simulink model "finalproject"  (R2022a)
settings: Solver=VariableStepAuto  StartTime=0.0  StopTime=0.1  RelTol=1e-3
values from neighbouring files (symbols this model uses):
  A_opamp = 2e5    (= 200000)    [flybackcode.m]
  C = 5e-3    (= 0.005)    [flybackcode.m]
  C1 = 25.6e-9    (= 2.56e-08)    [flybackcode.m]
  C2 = 3.02e-9    (= 3.02e-09)    [flybackcode.m]
  C3 = 4.4e-9    (= 4.4e-09)    [flybackcode.m]
  limit = 0.1    [flybackcode.m]
  R1 = 100e3    (= 100000)    [flybackcode.m]
  R2 = 18.918e3    (= 18918)    [flybackcode.m]
  R3 = 11.5e3    (= 11500)    [flybackcode.m]
  Ra = ((Vo/Vref) *Rb)- Rb    (= 400000)    [flybackcode.m]
  Rb = 100e3    (= 100000)    [flybackcode.m]
  Rin_opamp = 1e7    (= 10000000)    [flybackcode.m]
  RL = 2.05326    [flybackcode.m]
  Rout_opamp = 1e-3    (= 0.001)    [flybackcode.m]
  Vp = Vref/D    (= 5.90115564298)    [flybackcode.m]
  Vref = 2.4    [flybackcode.m]
libraries: spsSeriesRLCBranchLib x13, spsVoltageMeasurementLib x5, spsDCVoltageSourceLib x2, slctrlblks x1, spsCurrentMeasurementLib x1, spsDiodeLib x1, spsGroundLib x1, spsLinearTransformerLib x1, spsMosfetLib x1, spsSawtoothGeneratorLib x1, spsControlledVoltageSourceLib x1, spspowerguiLib x1
settings Model: Creator=justi  LastModifiedBy=justi

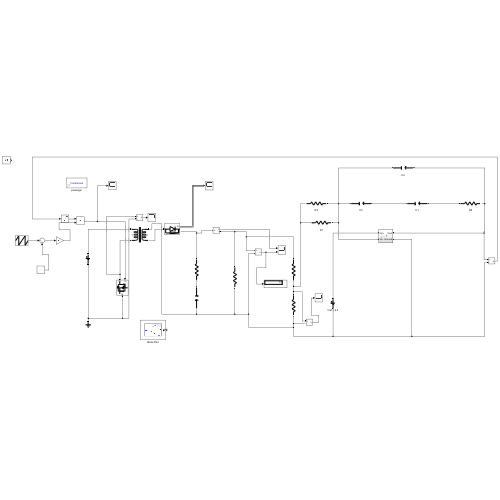
[thumbnail: Simulink's stored preview of the top-level diagram]
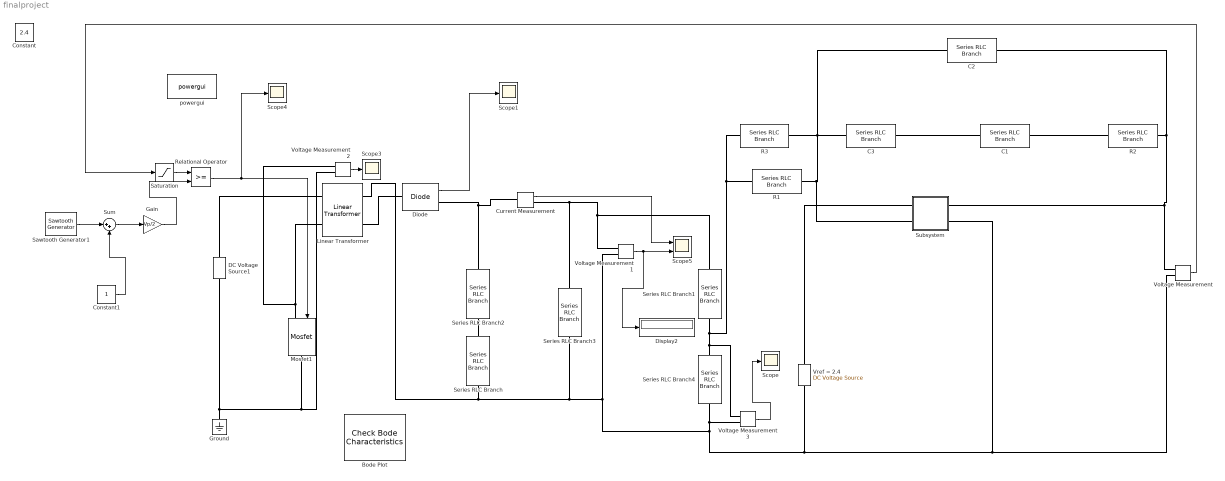
== system finalproject ==
  Bode Plot : slctrlblks/Model Verification/Check Bode  Characteristics  InstantiateOnLoad=on  SaveOperatingPoints=off  LinearizationIOs={'/Relational Operator', 1, 'in', 'off', '';'/Voltage Measurement1', 1, 'out', 'on', ''}  LinearizeAt=SnapshotTimes  SnapshotTimes=[0]  TriggerType=rising  SampleTime=auto  RateConversionMethod=zoh  PreWarpFreq=10  UseExactDelayModel=off  UseFullBlockNameLabels=off  UseBusSignalLabels=off  enabled=on  stopWhenAssertionFail=off  export=on  ViewDlgPos=[460 610 601 534]  OpenViewOnLoad=on  LaunchViewOnOpen=off  FrequencyUnits=rad/s  MagnitudeUnits=dB  PhaseUnits=deg  TimeUnits=seconds  EnableUpperBound=on  UpperBoundFrequencies=[]  UpperBoundMagnitudes=[]  EnableLowerBound=off  LowerBoundFrequencies=[]  LowerBoundMagnitudes=[]
      settings: SaveToWorkspace=on
  C1 : spsSeriesRLCBranchLib/Series RLC Branch  LConnTagsString=__new0  RConnTagsString=__new0  BranchType=C  Resistance=R3  Inductance=1e-3  SetiL0=off  InitialCurrent=0  Capacitance=C1  Setx0=off  InitialVoltage=0  Measurements=None
  C2 : spsSeriesRLCBranchLib/Series RLC Branch  LConnTagsString=__new0  RConnTagsString=__new0  BranchType=C  Resistance=R3  Inductance=1e-3  SetiL0=off  InitialCurrent=0  Capacitance=C2  Setx0=off  InitialVoltage=0  Measurements=None
  C3 : spsSeriesRLCBranchLib/Series RLC Branch  LConnTagsString=__new0  RConnTagsString=__new0  BranchType=C  Resistance=R3  Inductance=1e-3  SetiL0=off  InitialCurrent=0  Capacitance=C3  Setx0=off  InitialVoltage=0  Measurements=None
  Constant : Constant  Value=2.4
  Constant1 : Constant
  Current Measurement : spsCurrentMeasurementLib/Current Measurement  PhasorSimulation=off  OutputType=Complex  PSBequivalent=0
  DC Voltage Source1 : spsDCVoltageSourceLib/DC Voltage Source  Amplitude=70  Measurements=None
  Diode : spsDiodeLib/Diode  Ron=0.001  Lon=0  Vf=0.8  IC=0  UseSnubber=0  Rs=500  Cs=250e-9  Measurements=on
  Display2 : Display
  Gain : Gain  Gain=Vp/2
  Ground : spsGroundLib/Ground  LConnTagsString=a
  Linear Transformer : spsLinearTransformerLib/Linear Transformer  UNITS=SI  NominalPower=[ 250e6 100e3 ]  winding1=[280 0 0]  winding2=[70 0 0]  ThreeWindings=off  winding3=[3.15e+05 0.7938 0.084225]  RmLm=[1.0804e+05 100e-6]  Measurements=None  DataType=on
  Mosfet1 : spsMosfetLib/Mosfet  Ron=0.1  Lon=0  Rd=0  Vfd=0  IC=0  Rs=1e5  Cs=inf  Measurements=off
  R1 : spsSeriesRLCBranchLib/Series RLC Branch  LConnTagsString=__new0  RConnTagsString=__new0  BranchType=R  Resistance=R1  Inductance=1e-3  SetiL0=off  InitialCurrent=0  Capacitance=1e-6  Setx0=off  InitialVoltage=0  Measurements=None
  R2 : spsSeriesRLCBranchLib/Series RLC Branch  LConnTagsString=__new0  RConnTagsString=__new0  BranchType=R  Resistance=R2  Inductance=1e-3  SetiL0=off  InitialCurrent=0  Capacitance=1e-6  Setx0=off  InitialVoltage=0  Measurements=None
  R3 : spsSeriesRLCBranchLib/Series RLC Branch  LConnTagsString=__new0  RConnTagsString=__new0  BranchType=R  Resistance=R3  Inductance=1e-3  SetiL0=off  InitialCurrent=0  Capacitance=1e-6  Setx0=off  InitialVoltage=0  Measurements=None
  Relational Operator : RelationalOperator  OutDataTypeStr=boolean  RndMeth=Simplest  InputSameDT=off
  Saturation : Saturate  UpperLimit=Vp-limit  LowerLimit=0+limit
  Sawtooth Generator1 : spsSawtoothGeneratorLib/Sawtooth Generator  Freq=fsw  Phase=-180  Ts=0
  Scope{,1,3..4} (4 alike) : Scope
  Scope5 : Scope  NumInputPorts=2
  Series RLC Branch : spsSeriesRLCBranchLib/Series RLC Branch  LConnTagsString=__new0  RConnTagsString=__new0  BranchType=C  Resistance=1  Inductance=1e-3  SetiL0=off  InitialCurrent=0  Capacitance=5e-3  Setx0=on  InitialVoltage=0  Measurements=None
  Series RLC Branch1 : spsSeriesRLCBranchLib/Series RLC Branch  LConnTagsString=__new0  RConnTagsString=__new0  BranchType=R  Resistance=Ra  Inductance=1e-3  SetiL0=off  InitialCurrent=0  Capacitance=1e-6  Setx0=off  InitialVoltage=0  Measurements=None
  Series RLC Branch2 : spsSeriesRLCBranchLib/Series RLC Branch  LConnTagsString=__new0  RConnTagsString=__new0  BranchType=R  Resistance=1.0e-3  Inductance=1e-3  SetiL0=off  InitialCurrent=0  Capacitance=C  Setx0=on  InitialVoltage=0  Measurements=None
  Series RLC Branch3 : spsSeriesRLCBranchLib/Series RLC Branch  LConnTagsString=__new0  RConnTagsString=__new0  BranchType=R  Resistance=RL  Inductance=1e-3  SetiL0=off  InitialCurrent=0  Capacitance=0  Setx0=off  InitialVoltage=0  Measurements=None
  Series RLC Branch4 : spsSeriesRLCBranchLib/Series RLC Branch  LConnTagsString=__new0  RConnTagsString=__new0  BranchType=R  Resistance=Rb  Inductance=1e-3  SetiL0=off  InitialCurrent=0  Capacitance=1e-6  Setx0=off  InitialVoltage=0  Measurements=None
  Subsystem : Subsystem
  Sum : Sum  Inputs=|++
  Voltage Measurement{,1..3} (4 alike) : spsVoltageMeasurementLib/Voltage Measurement  PhasorSimulation=off  OutputType=Complex  PSBequivalent=0
  Vref = 2.4 : spsDCVoltageSourceLib/DC Voltage Source  Amplitude=Vref  Measurements=None
  powergui : spspowerguiLib/powergui  Priority=1  SimulationMode=Continuous  SampleTime=50e-6  frequency=60  Iterations=50  frequencyindice=0  Pbase=100e6  ErrMax=1e-4  UnitsV=kV  UnitsW=MW  buscounter=0  FunctionMessages=off  echomessages=off  EnableUseOfTLC=off  CurrentSourceSwitches=off  DisableSnubberDevices=off  DisableRonSwitches=on  DisableVfSwitches=on  DisplayEquations=off  AutomaticDiscreteSolvers=off  SolverType=Tustin/Backward Euler (TBE)  Interpol=off  ExternalGateDelay=off  methode=off  Ts=100  x0status=blocks  SPID=on  SwTol=0  HookPort=off  NonlinearTolerance=1e-4  nMaxIteration=100  ContinueOnMaxIteration=off  RestoreLinks=warning  ResistiveCurrentMeasurement=off  Frange=[0:2:500]  Ylog=off  Xlog=on  ShowGrid=off  save=off  variable=ZData  structure=0  ZoomFFT=off  StartTime=0.0  cycles=1  DisplayStyle=1  fundamental=60  FreqAxis=off  MaxFrequency=1000  frequencyindicesteady=1  RmsSteady=1  display=off
  wires:
  Voltage Measurement1/1 -> Display2/1, Scope5/2
  Constant1/1 -> Sum/2
  Sawtooth Generator1/1 -> Sum/1
  Sum/1 -> Gain/1
  Gain/1 -> Relational Operator/2
  Current Measurement/1 -> Scope5/1
  Voltage Measurement2/1 -> Scope3/1
  Relational Operator/1 -> Scope4/1, Mosfet1/1
  Voltage Measurement3/1 -> Scope/1
  Diode/1 -> Scope1/1
  Saturation/1 -> Relational Operator/1
  Voltage Measurement/1 -> Saturation/1
  connections:
  Series RLC Branch2/LConn1 -- Diode/RConn1 -- Current Measurement/LConn1
  Voltage Measurement2/LConn2 -- Mosfet1/RConn1 -- DC Voltage Source1/LConn1 -- Ground/LConn1
  C3/LConn1 -- Subsystem/LConn2 -- R1/RConn1 -- C2/LConn1 -- R3/RConn1
  C1/LConn1 -- C3/RConn1
  C1/RConn1 -- R2/LConn1
  Vref = 2.4/RConn1 -- Subsystem/LConn1
  C2/RConn1 -- Voltage Measurement/LConn1 -- Subsystem/RConn1 -- R2/RConn1
  Linear Transformer/LConn2 -- Mosfet1/LConn1 -- Voltage Measurement2/LConn1
  Linear Transformer/LConn1 -- DC Voltage Source1/RConn1
  Series RLC Branch/LConn1 -- Series RLC Branch2/RConn1
  Series RLC Branch1/RConn1 -- R3/LConn1 -- R1/LConn1 -- Voltage Measurement3/LConn1 -- Series RLC Branch4/LConn1
  Series RLC Branch1/LConn1 -- Series RLC Branch3/LConn1 -- Current Measurement/RConn1 -- Voltage Measurement1/LConn1
  Series RLC Branch3/RConn1 -- Subsystem/RConn2 -- Voltage Measurement/LConn2 -- Vref = 2.4/LConn1 -- Series RLC Branch4/RConn1 -- Voltage Measurement3/LConn2 -- Voltage Measurement1/LConn2 -- Series RLC Branch/RConn1 -- Linear Transformer/RConn1
  Linear Transformer/RConn2 -- Diode/LConn1

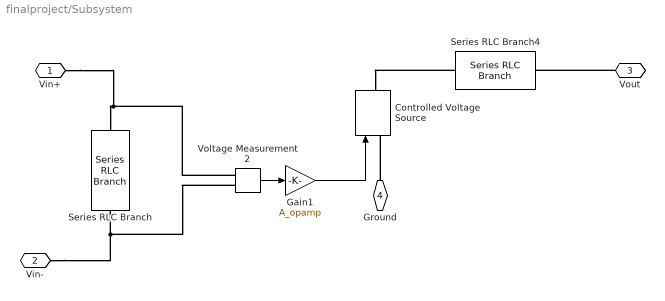
== system finalproject/Subsystem ==
  Controlled Voltage Source : spsControlledVoltageSourceLib/Controlled Voltage Source  Initialize=on  Source_Type=DC  Amplitude=0  Phase=0  Frequency=0  Measurements=None
  Gain1 : Gain  Gain=A_opamp
  Series RLC Branch : spsSeriesRLCBranchLib/Series RLC Branch  LConnTagsString=__new0  RConnTagsString=__new0  BranchType=R  Resistance=Rin_opamp  Inductance=1e-3  SetiL0=off  InitialCurrent=0  Capacitance=1e-6  Setx0=off  InitialVoltage=0  Measurements=None
  Series RLC Branch4 : spsSeriesRLCBranchLib/Series RLC Branch  LConnTagsString=__new0  RConnTagsString=__new0  BranchType=R  Resistance=Rout_opamp  Inductance=1e-3  SetiL0=off  InitialCurrent=0  Capacitance=1e-6  Setx0=off  InitialVoltage=0  Measurements=None
  Voltage Measurement2 : spsVoltageMeasurementLib/Voltage Measurement  PhasorSimulation=off  OutputType=Complex  PSBequivalent=0
  Vin+ : PMIOPort  Side=Left
  Vin- : PMIOPort  Port=2  Side=Left
  Vout : PMIOPort  Port=3  Side=Right
  Ground : PMIOPort  Port=4  Side=Right
  wires:
  Gain1/1 -> Controlled Voltage Source/1
  Voltage Measurement2/1 -> Gain1/1
  connections:
  Series RLC Branch4/RConn1 -- Controlled Voltage Source/RConn1
  Voltage Measurement2/LConn1 -- Vin+/RConn1 -- Series RLC Branch/RConn1
  Vout/RConn1 -- Series RLC Branch4/LConn1
  Ground/RConn1 -- Controlled Voltage Source/LConn1
  Voltage Measurement2/LConn2 -- Vin-/RConn1 -- Series RLC Branch/LConn1
